simulink model "DOF_14_Vehicle"  (R2018a)
settings: Solver=FixedStepDiscrete  StartTime=0.0  StopTime=inf  FixedStep=0.002  RelTol=1e-3  EnableMultiTasking=on
PreLoadFcn:
  | DOF_14_param
  | if exist('tl_preloadfcn','file'), tl_preloadfcn(gcs,403); end
PostLoadFcn:
  | if exist('tl_postloadfcn','file'), tl_postloadfcn(gcs,403); end
InitFcn:
  | DOF_14_param
  | if exist('tlds_init','file'), tlds_init(gcs); end
StartFcn:
  | if exist('tlds_start','file'), tlds_start(gcs); end
StopFcn:
  | if exist('tlds_stop','file'), tlds_stop(gcs); end
values from neighbouring files (symbols this model uses):
  mu = muf+mur    (= 160)    [DOF_14_param.m]
  ro = 0.285    [DOF_14_param.m]
  Ts = 0.001    [DOF_14_param.m]
PreSaveFcn:
  | if exist('tl_presavefcn','file'), tl_presavefcn(gcs); end
CloseFcn:
  | if exist('tl_closefcn','file'), tl_closefcn(gcs); end
settings Model: ExtModeTrigDuration=10000  Creator=srivats  LastModifiedBy=srivats
settings SolverCC: PositivePriorityOrder=on
settings RTWCC: SystemTargetFile=quarc_win64.tlc  TemplateMakefile=quarc_default_tmf  Description=QUARC Win64 Target
settings STFCustomTargetCC: TargetPreCompLibLocation=C:\PROGRA~3\QUARC\lib\2018a\win64\release  TargetLangStandard=C99 (ISO)  ConcurrentExecutionCompliant=on  SystemTargetFile=quarc_win64.tlc
settings GRTTargetCC: TargetPreCompLibLocation=C:\PROGRA~3\QUARC\lib\2018a\win64\release  ParMdlRefBuildCompliant=off  CompOptLevelCompliant=off  CombineOutputUpdateFcns=off  MatFileLogging=off  CPPClassGenCompliant=off  GRTInterface=on  UseToolchainInfoCompliant=off  ExtMode=on  ExtModeMexFile=quarc_comm

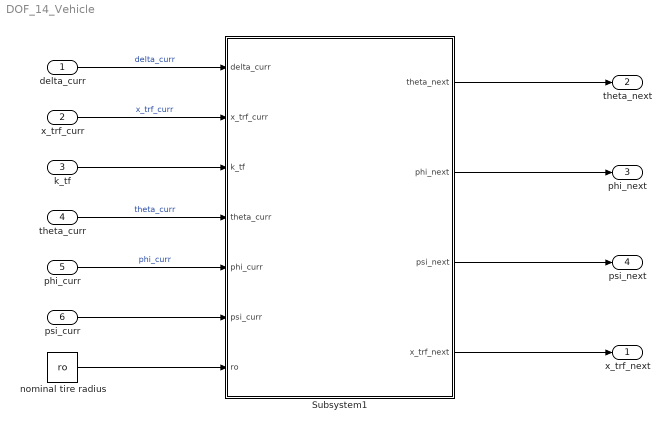
== system DOF_14_Vehicle ==
  delta_curr : Inport  SampleTime=Ts
  x_trf_curr : Inport  Port=2  SampleTime=Ts
  k_tf : Inport  Port=3  SampleTime=Ts
  theta_curr : Inport  Port=4  SampleTime=Ts
  phi_curr : Inport  Port=5  SampleTime=Ts
  psi_curr : Inport  Port=6  SampleTime=Ts
  Subsystem1 : Subsystem
  nominal tire radius : Constant  Value=ro
  x_trf_next : Outport  SampleTime=Ts
  theta_next : Outport  Port=2  SampleTime=Ts
  phi_next : Outport  Port=3  SampleTime=Ts
  psi_next : Outport  Port=4  SampleTime=Ts
  wires:
  delta_curr/1 -> Subsystem1/1(delta_curr)  "delta_curr"
  x_trf_curr/1 -> Subsystem1/2(x_trf_curr)  "x_trf_curr"
  k_tf/1 -> Subsystem1/3(k_tf)
  theta_curr/1 -> Subsystem1/4(theta_curr)  "theta_curr"
  phi_curr/1 -> Subsystem1/5(phi_curr)  "phi_curr"
  psi_curr/1 -> Subsystem1/6(psi_curr)
  Subsystem1/1(theta_next) -> theta_next/1
  Subsystem1/2(phi_next) -> phi_next/1
  Subsystem1/3(psi_next) -> psi_next/1
  Subsystem1/4(x_trf_next) -> x_trf_next/1
  nominal tire radius/1 -> Subsystem1/7(ro)

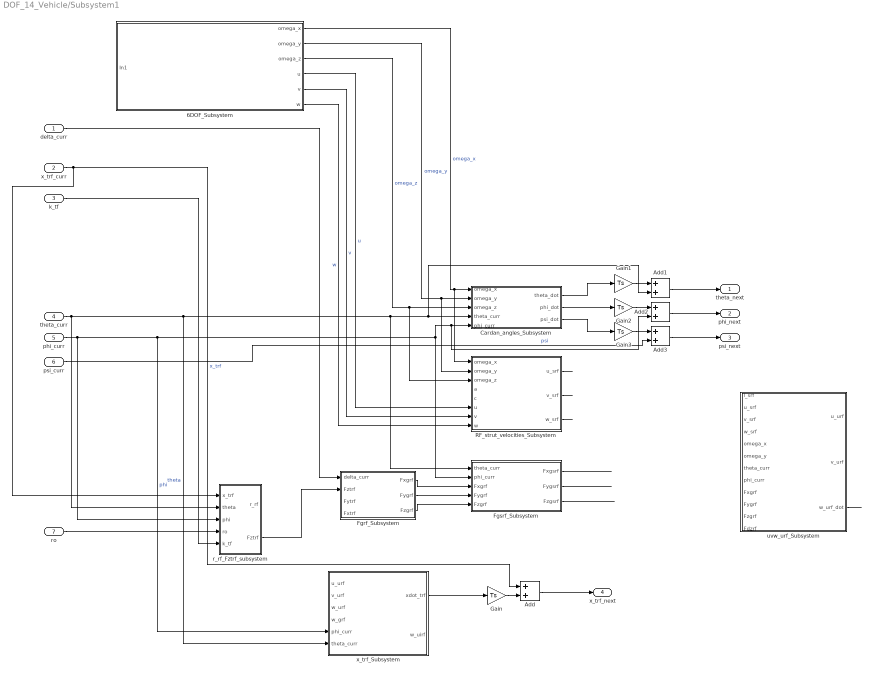
== system DOF_14_Vehicle/Subsystem1 ==
  delta_curr : Inport  SampleTime=Ts
  x_trf_curr : Inport  Port=2  SampleTime=Ts
  k_tf : Inport  Port=3  SampleTime=Ts
  theta_curr : Inport  Port=4  SampleTime=Ts
  phi_curr : Inport  Port=5  SampleTime=Ts
  psi_curr : Inport  Port=6  SampleTime=Ts
  ro : Inport  Port=7  SampleTime=Ts
  6DOF_Subsystem : Subsystem
  Add{,1..3} (4 alike) : Sum
  Cardan_angles_Subsystem : Subsystem
  Fgrf_Subsystem : Subsystem
  Fgsrf_Subsystem : Subsystem
  Gain{,1..3} (4 alike) : Gain  Gain=Ts
  RF_strut_velocities_Subsystem : Subsystem
  r_rf_Fztrf_subsystem : Subsystem
  uvw_urf_Subsystem : Subsystem
  x_trf_Subsystem : Subsystem
  theta_next : Outport  SampleTime=Ts
  phi_next : Outport  Port=2  SampleTime=Ts
  psi_next : Outport  Port=3  SampleTime=Ts
  x_trf_next : Outport  Port=4  SampleTime=Ts
  wires:
  psi_curr/1 -> Add3/2  "psi"
  Add2/1 -> phi_next/1
  6DOF_Subsystem/6(w) -> RF_strut_velocities_Subsystem/8(w)  "w"
  k_tf/1 -> r_rf_Fztrf_subsystem/5(k_tf)
  ? -> x_trf_Subsystem/4(w_grf)
  Fgrf_Subsystem/1(Fxgrf) -> Fgsrf_Subsystem/3(Fxgrf)
  x_trf_Subsystem/1(xdot_trf) -> Gain/1
  x_trf_curr/1 -> Add/1, r_rf_Fztrf_subsystem/1(x_trf)  "x_trf"
  Add/1 -> x_trf_next/1
  Add3/1 -> psi_next/1
  Cardan_angles_Subsystem/2(phi_dot) -> Gain2/1
  Add1/1 -> theta_next/1
  RF_strut_velocities_Subsystem/3(w_srf) -> ?
  Cardan_angles_Subsystem/1(theta_dot) -> Gain1/1
  Fgrf_Subsystem/2(Fygrf) -> Fgsrf_Subsystem/4(Fygrf)
  6DOF_Subsystem/2(omega_y) -> RF_strut_velocities_Subsystem/2(omega_y), Cardan_angles_Subsystem/2(omega_y)  "omega_y"
  Gain3/1 -> Add3/1
  phi_curr/1 -> r_rf_Fztrf_subsystem/3(phi), Add2/2, Cardan_angles_Subsystem/5(phi_curr), Fgsrf_Subsystem/2(phi_curr), x_trf_Subsystem/5(phi_curr)  "phi"
  Cardan_angles_Subsystem/3(psi_dot) -> Gain3/1
  ? -> Fgrf_Subsystem/3(Fytrf)
  Fgsrf_Subsystem/1(Fxgsrf) -> ?
  Gain1/1 -> Add1/1
  ? -> x_trf_Subsystem/3(w_urf)
  6DOF_Subsystem/5(v) -> RF_strut_velocities_Subsystem/7(v)  "v"
  Fgrf_Subsystem/3(Fzgrf) -> Fgsrf_Subsystem/5(Fzgrf)
  Gain2/1 -> Add2/1
  delta_curr/1 -> Fgrf_Subsystem/1(delta_curr)
  ? -> RF_strut_velocities_Subsystem/4(a)
  Fgsrf_Subsystem/3(Fzgsrf) -> ?
  6DOF_Subsystem/4(u) -> RF_strut_velocities_Subsystem/6(u)  "u"
  Gain/1 -> Add/2
  ? -> RF_strut_velocities_Subsystem/5(c)
  6DOF_Subsystem/1(omega_x) -> RF_strut_velocities_Subsystem/1(omega_x), Cardan_angles_Subsystem/1(omega_x)  "omega_x"
  RF_strut_velocities_Subsystem/1(u_srf) -> ?
  theta_curr/1 -> r_rf_Fztrf_subsystem/2(theta), Fgsrf_Subsystem/1(theta_curr), Add1/2, Cardan_angles_Subsystem/4(theta_curr), x_trf_Subsystem/6(theta_curr)  "theta"
  ? -> x_trf_Subsystem/1(u_urf)
  Fgsrf_Subsystem/2(Fygsrf) -> ?
  ? -> x_trf_Subsystem/2(v_urf)
  RF_strut_velocities_Subsystem/2(v_srf) -> ?
  6DOF_Subsystem/3(omega_z) -> RF_strut_velocities_Subsystem/3(omega_z), Cardan_angles_Subsystem/3(omega_z)  "omega_z"
  ro/1 -> r_rf_Fztrf_subsystem/4(ro)
  r_rf_Fztrf_subsystem/2(Fztrf) -> Fgrf_Subsystem/2(Fztrf)
  uvw_urf_Subsystem/3(w_urf_dot) -> ?

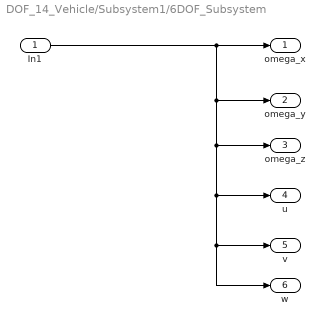
== system DOF_14_Vehicle/Subsystem1/6DOF_Subsystem ==
  In1 : Inport
  omega_x : Outport  SampleTime=Ts
  omega_y : Outport  Port=2  SampleTime=Ts
  omega_z : Outport  Port=3  SampleTime=Ts
  u : Outport  Port=4  SampleTime=Ts
  v : Outport  Port=5  SampleTime=Ts
  w : Outport  Port=6  SampleTime=Ts
  wires:
  In1/1 -> w/1, v/1, u/1, omega_z/1, omega_y/1, omega_x/1

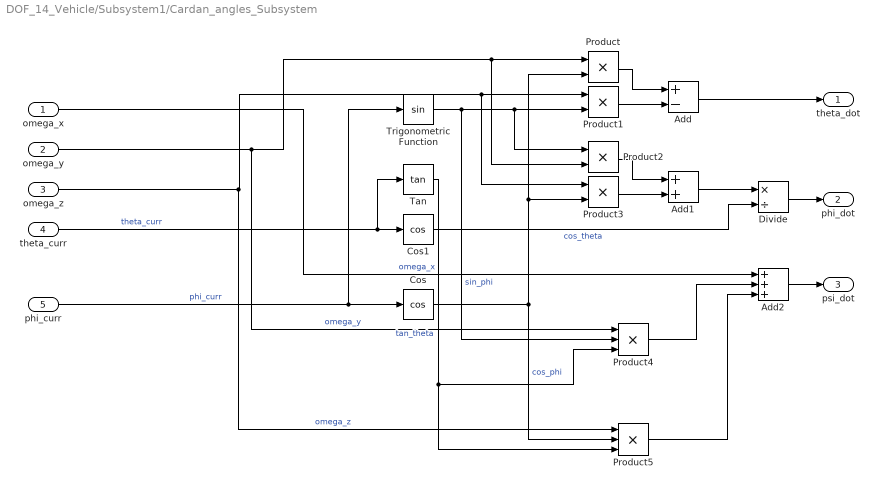
== system DOF_14_Vehicle/Subsystem1/Cardan_angles_Subsystem ==
  omega_x : Inport  SampleTime=Ts
  omega_y : Inport  Port=2  SampleTime=Ts
  omega_z : Inport  Port=3  SampleTime=Ts
  theta_curr : Inport  Port=4  SampleTime=Ts
  phi_curr : Inport  Port=5  SampleTime=Ts
  Add : Sum  Inputs=+-
  Add1 : Sum
  Add2 : Sum  Inputs=+++
  Cos : Trigonometry  Operator=cos
  Cos1 : Trigonometry  Operator=cos
  Divide : Product  Inputs=*/
  Product{,1..3} (4 alike) : Product
  Product4 : Product  Inputs=3
  Product5 : Product  Inputs=3
  Tan : Trigonometry  Operator=tan
  Trigonometric Function : Trigonometry
  theta_dot : Outport  SampleTime=Ts
  phi_dot : Outport  Port=2  SampleTime=Ts
  psi_dot : Outport  Port=3  SampleTime=Ts
  wires:
  omega_x/1 -> Add2/1  "omega_x"
  phi_curr/1 -> Trigonometric Function/1, Cos/1  "phi_curr"
  Cos/1 -> Product5/2, Product3/2, Product/2  "cos_phi"
  Add/1 -> theta_dot/1
  Product/1 -> Add/1
  omega_y/1 -> Product2/2, Product/1, Product4/1  "omega_y"
  Product1/1 -> Add/2
  Trigonometric Function/1 -> Product4/2, Product1/2, Product2/1  "sin_phi"
  omega_z/1 -> Product5/1, Product3/1, Product1/1  "omega_z"
  theta_curr/1 -> Tan/1, Cos1/1  "theta_curr"
  Product3/1 -> Add1/2
  Product2/1 -> Add1/1
  Add1/1 -> Divide/1
  Cos1/1 -> Divide/2  "cos_theta"
  Divide/1 -> phi_dot/1
  Add2/1 -> psi_dot/1
  Product4/1 -> Add2/2
  Tan/1 -> Product5/3, Product4/3  "tan_theta"
  Product5/1 -> Add2/3

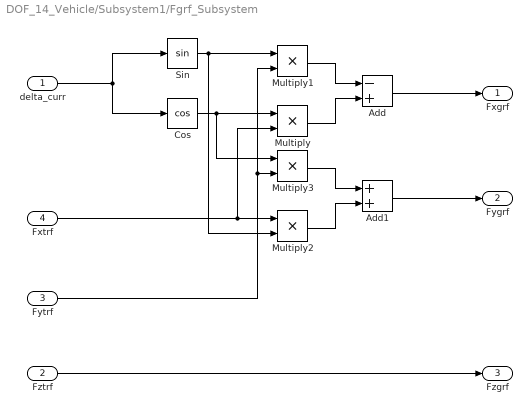
== system DOF_14_Vehicle/Subsystem1/Fgrf_Subsystem ==
  delta_curr : Inport  SampleTime=Ts
  Fztrf : Inport  Port=2  SampleTime=Ts
  Fytrf : Inport  Port=3  SampleTime=Ts
  Fxtrf : Inport  Port=4  SampleTime=Ts
  Add : Sum  Inputs=-+
  Add1 : Sum
  Cos : Trigonometry  Operator=cos
  Multiply{,1..3} (4 alike) : Product
  Sin : Trigonometry
  Fxgrf : Outport  SampleTime=Ts
  Fygrf : Outport  Port=2  SampleTime=Ts
  Fzgrf : Outport  Port=3  SampleTime=Ts
  wires:
  Fztrf/1 -> Fzgrf/1
  delta_curr/1 -> Cos/1, Sin/1
  Sin/1 -> Multiply2/2, Multiply1/1
  Cos/1 -> Multiply3/1, Multiply/1
  Fxtrf/1 -> Multiply2/1, Multiply/2
  Multiply/1 -> Add/2
  Fytrf/1 -> Multiply3/2, Multiply1/2
  Multiply1/1 -> Add/1
  Add/1 -> Fxgrf/1
  Multiply3/1 -> Add1/1
  Multiply2/1 -> Add1/2
  Add1/1 -> Fygrf/1

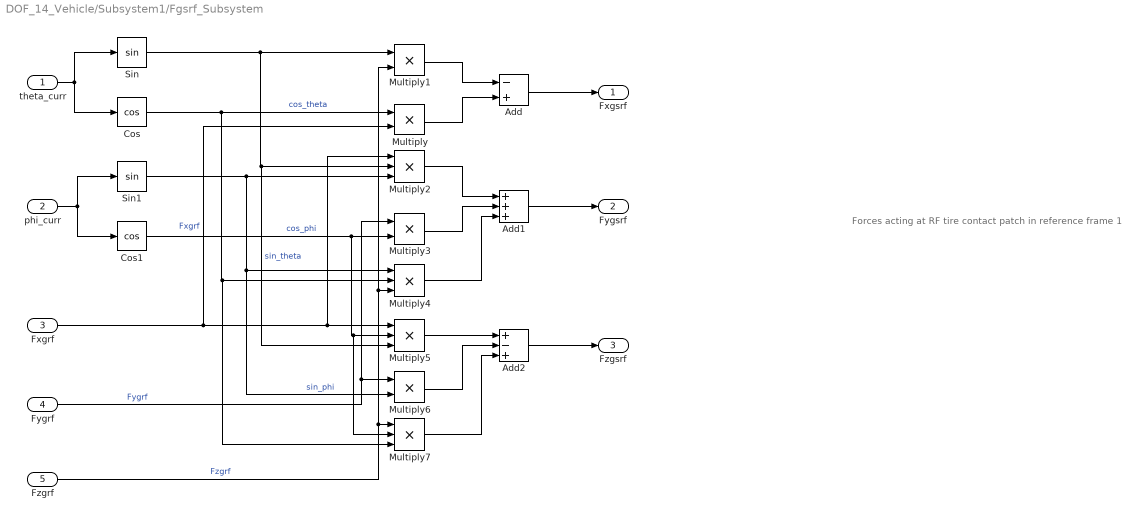
== system DOF_14_Vehicle/Subsystem1/Fgsrf_Subsystem ==
  note: Forces acting at RF tire contact patch in reference frame 1
  theta_curr : Inport  SampleTime=Ts
  phi_curr : Inport  Port=2  SampleTime=Ts
  Fxgrf : Inport  Port=3  SampleTime=Ts
  Fygrf : Inport  Port=4  SampleTime=Ts
  Fzgrf : Inport  Port=5  SampleTime=Ts
  Add : Sum  Inputs=-+
  Add1 : Sum  Inputs=+++
  Add2 : Sum  Inputs=+-+
  Cos : Trigonometry  Operator=cos
  Cos1 : Trigonometry  Operator=cos
  Multiply{,1,3,6} (4 alike) : Product
  Multiply{2,4..5,7} (4 alike) : Product  Inputs=3
  Sin : Trigonometry
  Sin1 : Trigonometry
  Fxgsrf : Outport  SampleTime=Ts
  Fygsrf : Outport  Port=2  SampleTime=Ts
  Fzgsrf : Outport  Port=3  SampleTime=Ts
  wires:
  phi_curr/1 -> Cos1/1, Sin1/1
  theta_curr/1 -> Cos/1, Sin/1
  Sin/1 -> Multiply5/3, Multiply2/2, Multiply1/1  "sin_theta"
  Cos/1 -> Multiply7/3, Multiply4/2, Multiply/1  "cos_theta"
  Sin1/1 -> Multiply6/2, Multiply4/1, Multiply2/3  "sin_phi"
  Cos1/1 -> Multiply7/2, Multiply5/2, Multiply3/2  "cos_phi"
  Fxgrf/1 -> Multiply/2, Multiply5/1, Multiply2/1  "Fxgrf"
  Fygrf/1 -> Multiply6/1, Multiply3/1  "Fygrf"
  Fzgrf/1 -> Multiply7/1, Multiply4/3, Multiply1/2  "Fzgrf"
  Multiply/1 -> Add/2
  Multiply1/1 -> Add/1
  Add/1 -> Fxgsrf/1
  Multiply2/1 -> Add1/1
  Multiply3/1 -> Add1/2
  Multiply4/1 -> Add1/3
  Add1/1 -> Fygsrf/1
  Multiply5/1 -> Add2/1
  Multiply6/1 -> Add2/2
  Multiply7/1 -> Add2/3
  Add2/1 -> Fzgsrf/1

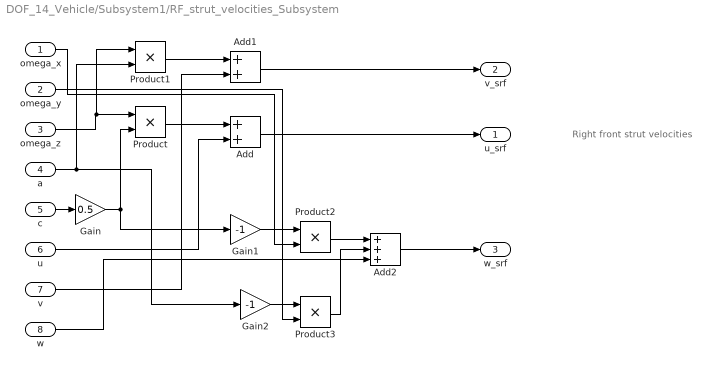
== system DOF_14_Vehicle/Subsystem1/RF_strut_velocities_Subsystem ==
  note: Right front strut velocities
  omega_x : Inport  SampleTime=Ts
  omega_y : Inport  Port=2  SampleTime=Ts
  omega_z : Inport  Port=3  SampleTime=Ts
  a : Inport  Port=4  SampleTime=Ts
  c : Inport  Port=5  SampleTime=Ts
  u : Inport  Port=6  SampleTime=Ts
  v : Inport  Port=7  SampleTime=Ts
  w : Inport  Port=8  SampleTime=Ts
  Add : Sum
  Add1 : Sum
  Add2 : Sum  Inputs=+++
  Gain : Gain  Gain=0.5
  Gain1 : Gain  Gain=-1
  Gain2 : Gain  Gain=-1
  Product{,1..3} (4 alike) : Product
  u_srf : Outport  SampleTime=Ts
  v_srf : Outport  Port=2  SampleTime=Ts
  w_srf : Outport  Port=3  SampleTime=Ts
  wires:
  Product/1 -> Add/1
  omega_z/1 -> Product1/1, Product/1
  c/1 -> Gain/1
  Gain/1 -> Gain1/1, Product/2
  u/1 -> Add/2
  Add/1 -> u_srf/1
  Product1/1 -> Add1/1
  Add1/1 -> v_srf/1
  a/1 -> Gain2/1, Product1/2
  v/1 -> Add1/2
  Gain1/1 -> Product2/1
  omega_x/1 -> Product2/2
  Gain2/1 -> Product3/1
  omega_y/1 -> Product3/2
  Product2/1 -> Add2/1
  Product3/1 -> Add2/2
  w/1 -> Add2/3
  Add2/1 -> w_srf/1

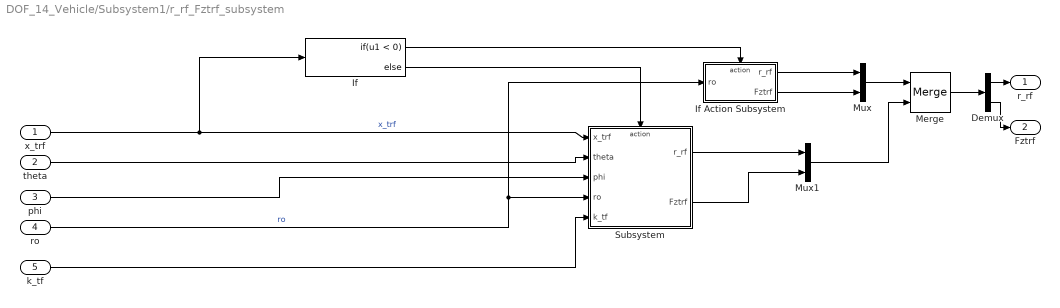
== system DOF_14_Vehicle/Subsystem1/r_rf_Fztrf_subsystem ==
  x_trf : Inport
  theta : Inport  Port=2
  phi : Inport  Port=3
  ro : Inport  Port=4  SampleTime=Ts
  k_tf : Inport  Port=5
  Demux : Demux  Outputs=2
  If : If  IfExpression=u1 < 0
  If Action Subsystem : Subsystem  TreatAsAtomicUnit=on
  Merge : Merge
  Mux : Mux  Inputs=2
  Mux1 : Mux  Inputs=2
  Subsystem : Subsystem
  r_rf : Outport
  Fztrf : Outport  Port=2
  wires:
  x_trf/1 -> If/1, Subsystem/1(x_trf)  "x_trf"
  ro/1 -> If Action Subsystem/1(ro), Subsystem/4(ro)  "ro"
  If/1 -> If Action Subsystem/Action
  theta/1 -> Subsystem/2(theta)
  phi/1 -> Subsystem/3(phi)
  Subsystem/1(r_rf) -> Mux1/1
  If/2 -> Subsystem/Action
  If Action Subsystem/1(r_rf) -> Mux/1
  If Action Subsystem/2(Fztrf) -> Mux/2
  k_tf/1 -> Subsystem/5(k_tf)
  Subsystem/2(Fztrf) -> Mux1/2
  Mux/1 -> Merge/1
  Mux1/1 -> Merge/2
  Merge/1 -> Demux/1
  Demux/1 -> r_rf/1
  Demux/2 -> Fztrf/1

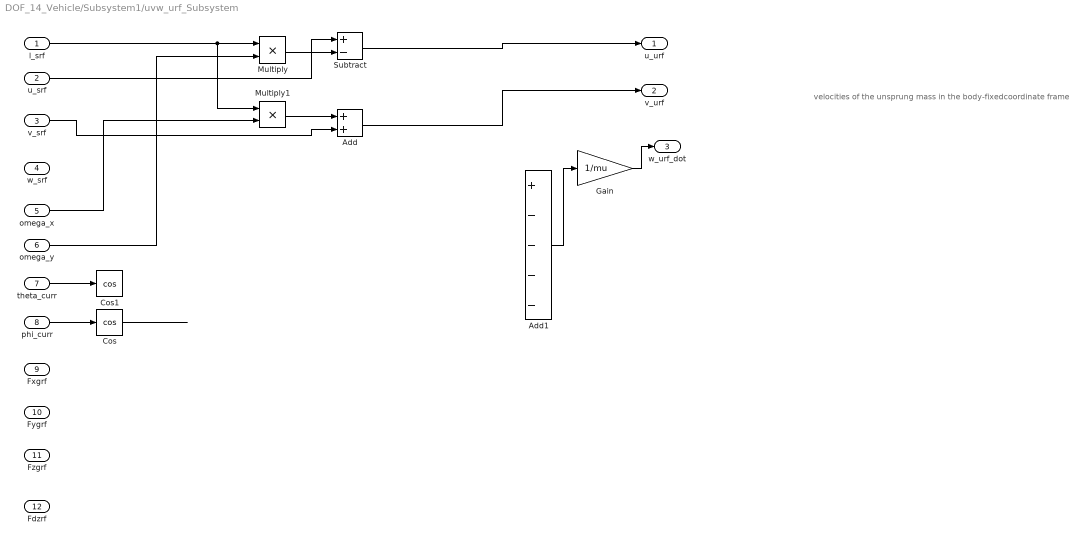
== system DOF_14_Vehicle/Subsystem1/uvw_urf_Subsystem ==
  note: velocities of the unsprung mass in the body-fixedcoordinate frame
  l_srf : Inport  SampleTime=Ts
  u_srf : Inport  Port=2  SampleTime=Ts
  v_srf : Inport  Port=3  SampleTime=Ts
  w_srf : Inport  Port=4  SampleTime=Ts
  omega_x : Inport  Port=5  SampleTime=Ts
  omega_y : Inport  Port=6  SampleTime=Ts
  theta_curr : Inport  Port=7  SampleTime=Ts
  phi_curr : Inport  Port=8  SampleTime=Ts
  Fxgrf : Inport  Port=9  SampleTime=Ts
  Fygrf : Inport  Port=10  SampleTime=Ts
  Fzgrf : Inport  Port=11  SampleTime=Ts
  Fdzrf : Inport  Port=12  SampleTime=Ts
  Add : Sum
  Add1 : Sum  Inputs=+----
  Cos : Trigonometry  Operator=cos
  Cos1 : Trigonometry  Operator=cos
  Gain : Gain  Gain=1/mu
  Multiply : Product
  Multiply1 : Product
  Subtract : Sum  Inputs=+-
  u_urf : Outport  SampleTime=Ts
  v_urf : Outport  Port=2  SampleTime=Ts
  w_urf_dot : Outport  Port=3  SampleTime=Ts
  wires:
  l_srf/1 -> Multiply1/1, Multiply/1
  omega_y/1 -> Multiply/2
  Multiply/1 -> Subtract/2
  u_srf/1 -> Subtract/1
  Subtract/1 -> u_urf/1
  omega_x/1 -> Multiply1/2
  Multiply1/1 -> Add/1
  v_srf/1 -> Add/2
  Add/1 -> v_urf/1
  Gain/1 -> w_urf_dot/1
  Add1/1 -> Gain/1
  phi_curr/1 -> Cos/1
  theta_curr/1 -> Cos1/1
  Cos/1 -> ?

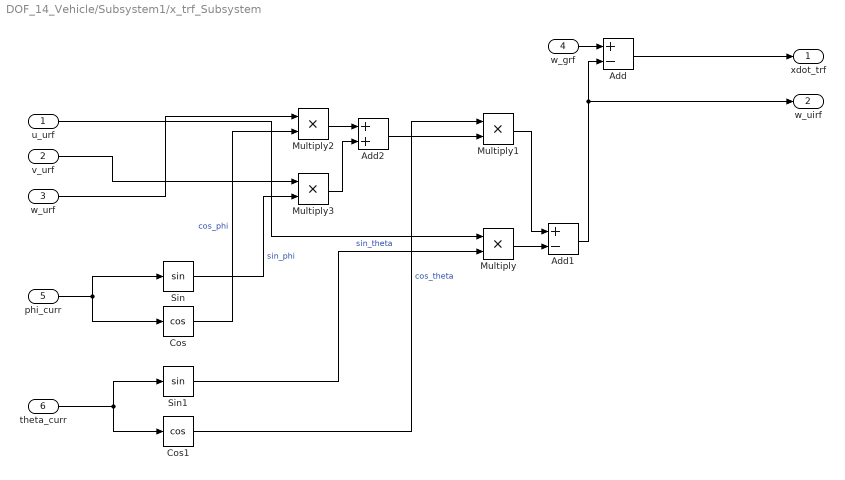
== system DOF_14_Vehicle/Subsystem1/x_trf_Subsystem ==
  u_urf : Inport  SampleTime=Ts
  v_urf : Inport  Port=2  SampleTime=Ts
  w_urf : Inport  Port=3  SampleTime=Ts
  w_grf : Inport  Port=4  SampleTime=Ts
  phi_curr : Inport  Port=5  SampleTime=Ts
  theta_curr : Inport  Port=6  SampleTime=Ts
  Add : Sum  Inputs=+-
  Add1 : Sum  Inputs=+-
  Add2 : Sum
  Cos : Trigonometry  Operator=cos
  Cos1 : Trigonometry  Operator=cos
  Multiply{,1..3} (4 alike) : Product
  Sin : Trigonometry
  Sin1 : Trigonometry
  xdot_trf : Outport  SampleTime=Ts
  w_uirf : Outport  Port=2  SampleTime=Ts
  wires:
  phi_curr/1 -> Sin/1, Cos/1
  theta_curr/1 -> Cos1/1, Sin1/1
  Sin/1 -> Multiply3/2  "sin_phi"
  Cos/1 -> Multiply2/2  "cos_phi"
  Sin1/1 -> Multiply/2  "sin_theta"
  Cos1/1 -> Multiply1/1  "cos_theta"
  w_grf/1 -> Add/1
  Add1/1 -> w_uirf/1, Add/2
  u_urf/1 -> Multiply/1
  Multiply/1 -> Add1/2
  Multiply1/1 -> Add1/1
  Add2/1 -> Multiply1/2
  Multiply2/1 -> Add2/1
  w_urf/1 -> Multiply2/1
  Multiply3/1 -> Add2/2
  v_urf/1 -> Multiply3/1
  Add/1 -> xdot_trf/1

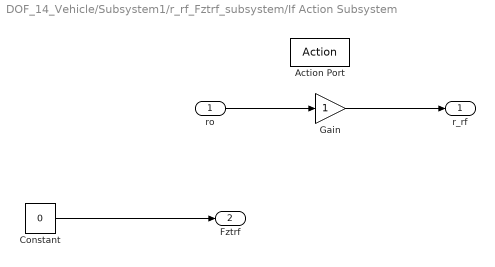
== system DOF_14_Vehicle/Subsystem1/r_rf_Fztrf_subsystem/If Action Subsystem ==
  ro : Inport
  Action Port : ActionPort  ActionType=then
  Constant : Constant  Value=0
  Gain : Gain
  r_rf : Outport
  Fztrf : Outport  Port=2
  wires:
  ro/1 -> Gain/1
  Gain/1 -> r_rf/1
  Constant/1 -> Fztrf/1

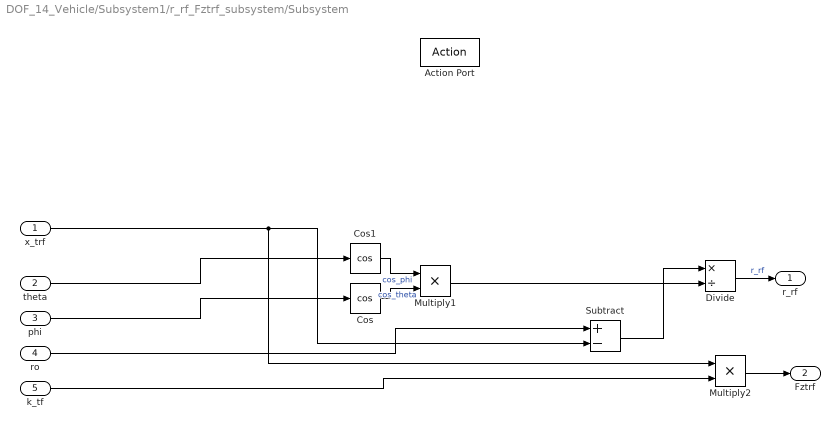
== system DOF_14_Vehicle/Subsystem1/r_rf_Fztrf_subsystem/Subsystem ==
  x_trf : Inport
  theta : Inport  Port=2
  phi : Inport  Port=3
  ro : Inport  Port=4
  k_tf : Inport  Port=5
  Action Port : ActionPort  ActionType=else
  Cos : Trigonometry  Operator=cos
  Cos1 : Trigonometry  Operator=cos
  Divide : Product  Inputs=*/
  Multiply1 : Product
  Multiply2 : Product
  Subtract : Sum  Inputs=+-
  r_rf : Outport
  Fztrf : Outport  Port=2
  wires:
  Cos1/1 -> Multiply1/1  "cos_phi"
  phi/1 -> Cos/1
  x_trf/1 -> Multiply2/1, Subtract/2
  Multiply1/1 -> Divide/2
  ro/1 -> Subtract/1
  Divide/1 -> r_rf/1  "r_rf"
  Subtract/1 -> Divide/1
  theta/1 -> Cos1/1
  Cos/1 -> Multiply1/2  "cos_theta"
  Multiply2/1 -> Fztrf/1
  k_tf/1 -> Multiply2/2
